simulink model "readFile"  (R2020a)
settings: Solver=VariableStepAuto  StartTime=0.0  StopTime=1440  RelTol=1e-3
settings Model: Creator=ramaz  LastModifiedBy=ramaz

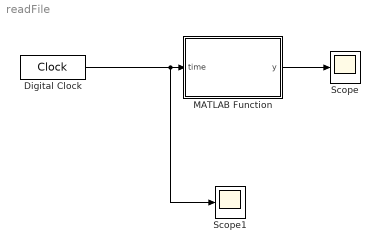
== system readFile ==
  Digital Clock : DigitalClock
  MATLAB Function : MATLAB Function  TreatAsAtomicUnit=on
  Scope : Scope
  Scope1 : Scope
  wires:
  Digital Clock/1 -> Scope1/1, MATLAB Function/1(time)
  MATLAB Function/1(y) -> Scope/1

== matlab function readFile/MATLAB Function ==
  data: time input; y output
function y = fcn(time)
    file = fopen('C:\\Users\\ramaz\\Desktop\\Bitirme_Projesi\\microgrid_matlab\\house1\\house_1_consume_power_1.txt','r');
    formatSpec = '%d';
    x = fscanf(file,formatSpec);
    if time == 0
        y = 0;
    elseif floor(time) == time
        y = x(time);
    else
        if floor(time) ~= 0
            y = x(floor(time));
        else
            y = 0;
        end
    end
    fclose(file);
end
